simulink model "moban1"  (R2022b)
settings: Solver=VariableStepAuto  StartTime=0.0  StopTime=4  RelTol=1e-3
InitFcn:
  | clear all;
  | 
  | Step_time=2;  %并网转离网的切换时间
  | Tf=0.0159*0.25 %直流侧电流滤波常数
  | 
  | Vdc_H2=720;   %直流母线电压最大值
  | Vdc_H1=710;   %
  | Udc=700;   %直流母线电压最大值
  | Vdc_L1=690;
  | Vdc_L2=680;   %直流母线电压最小值
  | 
  | %% 并网变流器部分 %%
  | P_grid=100e3;  %变流器额定功率
  | Cg=3227e-6;   %直流母线电容
  | P_grid=100e3;  %变流器额定功率
  | Idc_max=145;   %直流侧最大输出电流
  | %Rg=(720-700)/Idc_max;   %下垂系数
  | Rg=40*(Udc-40)/P_grid;   %下垂系数
  | Igrid_max=72;   %并网逆变器最大充放电电流（交流侧）
  | 
  | %% 蓄电池部分 %%
  | P_ba=50e3;  %变流器额定功率
  | R_ba=40*(Udc-40)/P_ba;
  | %Idc_max_ba=147;   %直流侧最大输出电流
  | %R_ba=(Vdc_L1-Vdc_L2)/P_ba;   %下垂系数
  | Iba_max=50;   %蓄电池恒流充放电电流
  | 
  | %% 光伏部分 %%
  | P_PV=150e3;  %变流器额定功率
  | R_PV=40*(Udc-40)/P_PV;   %下垂系数
  | Idc_max_PV=147;   %直流侧最大输出电流
model workspace (MAT data in the model file):
  C = 0.002
  GP = 1
  GQ = 0.01
  J = 5
  KQ = 0.06
  Kf = 800
  Kv = 577
  L = 0.002
  Ts = 5e-05
  Vdc = 400
  fsw = 20000
  wn = 314.159265359
undefined symbols (not defined in the file): DiscIntNeverNeededParam, Ion, Lithium, sigbuilder_block
libraries: spsCurrentMeasurementLib x8, spsSeriesRLCBranchLib x6, slpidlib x6, spsDiodeLib x4, spsVoltageMeasurementLib x3, spsFirstOrderFilterLib x3, spsabctodq0Lib x3, spsIGBTLib x3, spsThreePhaseSeriesRLCBranchLib x2, spsThreePhaseVIMeasurementLib x2, simulink x2, spsPower3phInstantaneousLib x1
(part 1 of 2)
settings Model: Creator=匡磊  LastModifiedBy=刘明炜
settings DataIOCC: ReturnWorkspaceOutputs=off

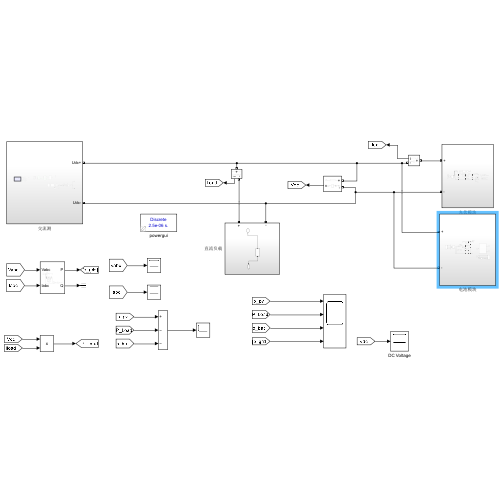
[thumbnail: Simulink's stored preview of the top-level diagram]
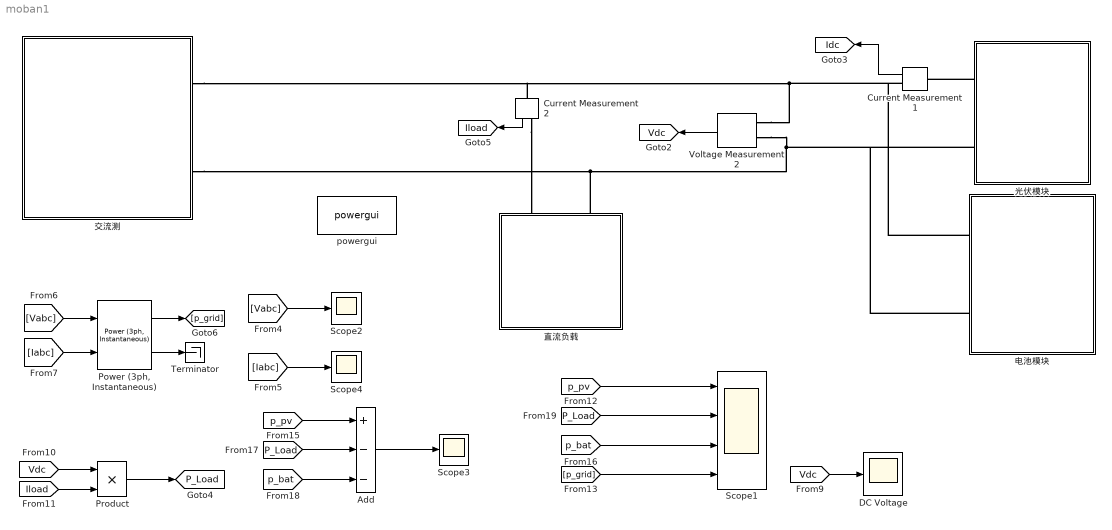
== system moban1 ==
  Add : Sum  Inputs=+--
  Current Measurement1 : spsCurrentMeasurementLib/Current Measurement  PhasorSimulation=off  OutputType=Complex  PSBequivalent=0
  Current Measurement2 : spsCurrentMeasurementLib/Current Measurement  PhasorSimulation=off  OutputType=Complex  PSBequivalent=0
  DC Voltage : Scope
  "Power (3ph, Instantaneous)" : spsPower3phInstantaneousLib/Power (3ph, Instantaneous)
  Product : Product
  Scope1 : Scope  NumInputPorts=4
  Scope2 : Scope
  Scope3 : Scope
  Scope4 : Scope
  Terminator : Terminator
  Voltage Measurement2 : spsVoltageMeasurementLib/Voltage Measurement  PhasorSimulation=off  OutputType=Complex  PSBequivalent=0
  powergui : spspowerguiLib/powergui  Priority=1  SimulationMode=Discrete  SampleTime=2.5e-6  frequency=60  Iterations=50  frequencyindice=0  Pbase=100e6  ErrMax=1e-4  UnitsV=kV  UnitsW=MW  buscounter=0  FunctionMessages=off  echomessages=off  EnableUseOfTLC=off  CurrentSourceSwitches=off  DisableSnubberDevices=off  DisableRonSwitches=off  DisableVfSwitches=off  DisplayEquations=off  AutomaticDiscreteSolvers=off  SolverType=Tustin/Backward Euler (TBE)  Interpol=off  ExternalGateDelay=off  methode=off  Ts=100  x0status=blocks  SPID=on  SwTol=0  HookPort=off  NonlinearTolerance=1e-4  nMaxIteration=100  ContinueOnMaxIteration=off  RestoreLinks=warning  ResistiveCurrentMeasurement=off  Frange=[0:2:500]  Ylog=off  Xlog=on  ShowGrid=off  save=off  variable=ZData  structure=0  ZoomFFT=off  StartTime=0.0  cycles=1  DisplayStyle=1  fundamental=60  FreqAxis=off  MaxFrequency=1000  frequencyindicesteady=1  RmsSteady=1  display=off
  交流测 : Subsystem
  光伏模块 : Subsystem
  电池模块 : Subsystem
  直流负载 : Subsystem
  tag scope: Idc=global, Iload=global, P_Load=global, Vdc=global
  wires:
  [p_pv] -> Scope1/1
  "Power (3ph, Instantaneous)"/1 -> [p_grid]
  [P_Load] -> Scope1/2
  [p_grid] -> Scope1/4
  Add/1 -> Scope3/1
  Current Measurement1/1 -> [Idc]
  [P_Load] -> Add/2
  [p_bat] -> Add/3
  [Vdc] -> DC Voltage/1
  Voltage Measurement2/1 -> [Vdc]
  [Vabc] -> "Power (3ph, Instantaneous)"/1
  [Vdc] -> Product/1
  [Iload] -> Product/2
  [p_pv] -> Add/1
  Product/1 -> [P_Load]
  Current Measurement2/1 -> [Iload]
  [p_bat] -> Scope1/3
  "Power (3ph, Instantaneous)"/2 -> Terminator/1
  [Iabc] -> "Power (3ph, Instantaneous)"/2
  [Vabc] -> Scope2/1
  [Iabc] -> Scope4/1
  connections:
  Voltage Measurement2/LConn1 -- Current Measurement2/LConn1 -- 交流测/LConn1 -- 电池模块/LConn1 -- Current Measurement1/RConn1
  交流测/LConn2 -- 直流负载/LConn2 -- 电池模块/LConn2 -- 光伏模块/LConn2 -- Voltage Measurement2/LConn2
  光伏模块/LConn1 -- Current Measurement1/LConn1
  Current Measurement2/RConn1 -- 直流负载/LConn1

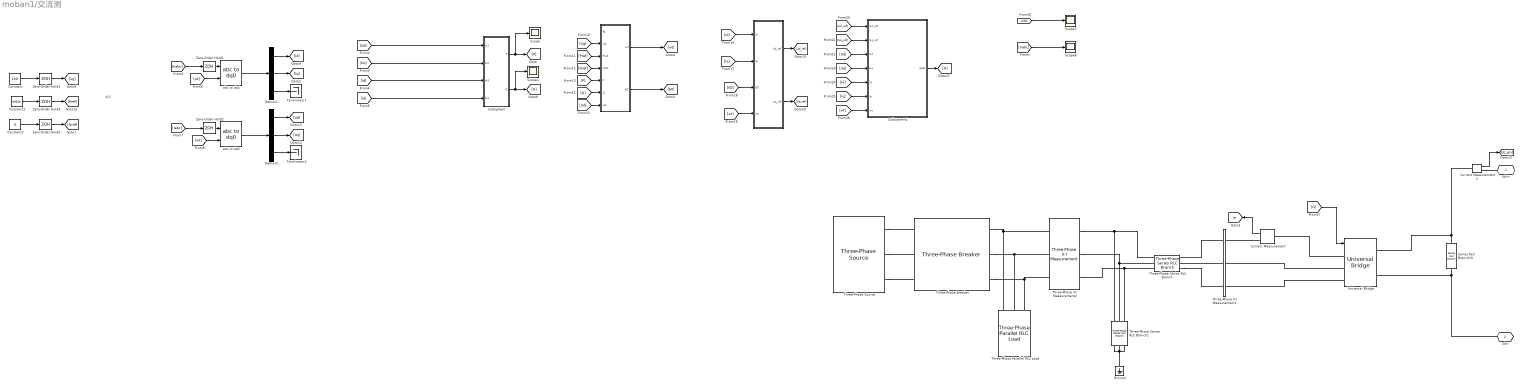
== system moban1/交流测 ==
  note: 给定
  "  " : Subsystem
  "   " : Subsystem
  Constant : Constant  Value=150
  Constant1 : Constant  Value=50000
  Constant2 : Constant  Value=0
  Current Measurement : spsCurrentMeasurementLib/Current Measurement  PhasorSimulation=off  OutputType=Complex  PSBequivalent=0
  Current Measurement1 : spsCurrentMeasurementLib/Current Measurement  PhasorSimulation=off  OutputType=Complex  PSBequivalent=0
  Demux1 : Demux  Outputs=3
  Demux2 : Demux  Outputs=3
  Ground : spsGroundLib/Ground  LConnTagsString=a
  Scope{,1,6..7} (4 alike) : Scope
  Series RLC Branch10 : spsSeriesRLCBranchLib/Series RLC Branch  LConnTagsString=__new0  RConnTagsString=__new0  BranchType=C  Resistance=0.001  Inductance=1e-3  SetiL0=off  InitialCurrent=0  Capacitance=Cg  Setx0=off  InitialVoltage=700  Measurements=None
  Subsystem : Subsystem
  Subsystem1 : Subsystem
  Terminator1 : Terminator
  Terminator2 : Terminator
  Three-Phase Parallel RLC Load : spsThreePhaseParallelRLCLoadLib/Three-Phase Parallel RLC Load  LConnTagsString=A|B|C  RConnTagsString=N  Configuration=Y (neutral)  NominalVoltage=380  Vabc=[1e3 1e3 1e3]  Vabcp=[1e3 1e3 1e3]  NominalFrequency=50  UnbalancedPower=off  ActivePower=50e3  InductivePower=0  CapacitivePower=0  Pabc=[10e3 9e3 11e3]  QLabc=[100 90 110]  QCabc=[100 90 110]  Pabcp=[10e3 9e3 11e3]  QLabcp=[100 90 110]  QCabcp=[100 90 110]  Measurements=None  LoadType=constant Z
  Three-Phase Series RLC Branch : spsThreePhaseSeriesRLCBranchLib/Three-Phase Series RLC Branch  LConnTagsString=A|B|C  RConnTagsString=A|B|C  BranchType=RL  Resistance=0  Inductance=7e-3  Capacitance=1e-6  Measurements=None
  Three-Phase Series RLC Branch1 : spsThreePhaseSeriesRLCBranchLib/Three-Phase Series RLC Branch  LConnTagsString=A|B|C  RConnTagsString=A|B|C  BranchType=RC  Resistance=1  Inductance=7e-3  Capacitance=1500e-6  Measurements=None
  Three-Phase V-I Measurement1 : spsThreePhaseVIMeasurementLib/Three-Phase V-I Measurement  VoltageMeasurement=no  SetLabelV=on  LabelV=Vabc  Vpu=off  VpuLL=off  CurrentMeasurement=yes  SetLabelI=on  LabelI=Iabc  Ipu=off  Pbase=100e6  Vbase=500e3  OutputType=Complex  PhasorSimulation=off  PSBequivalent=0
  Three-Phase V-I Measurement2 : spsThreePhaseVIMeasurementLib/Three-Phase V-I Measurement  VoltageMeasurement=phase-to-ground  SetLabelV=on  LabelV=Vabc  Vpu=off  VpuLL=off  CurrentMeasurement=no  SetLabelI=off  LabelI=Iabc1  Ipu=off  Pbase=100e6  Vbase=500e3  OutputType=Complex  PhasorSimulation=off  PSBequivalent=0
  Three-Phase Breaker : spsThreePhaseBreakerLib/Three-Phase Breaker  InitialState=closed  SwitchA=on  SwitchB=on  SwitchC=on  SwitchTimes=[1 1.5]  External=off  BreakerResistance=0.001  SnubberResistance=10e5  SnubberCapacitance=inf  Measurements=None
  Three-Phase Source : spsThreePhaseSourceLib/Three-Phase Source  InternalConnection=Y  VoltagePhases=off  Voltage=380  PhaseAngle=0  Voltage_phases=[25e3 25e3 25e3]/sqrt(3)  PhaseAngles_phases=[0 -120 +120]  Frequency=50  NonIdealSource=on  SpecifyImpedance=off  Resistance=0.001e-3  Inductance=0.001e-9  ShortCircuitLevel=100e6  BaseVoltage=380  XRratio=7  BusType=swing  Pref=10e3  Qref=0  Prefabc=[10e3, 10e3, 10e3]  Qrefabc=[0, 0, 0]  Qmin=-inf  Qmax=inf
  Universal Bridge : spsUniversalBridgeLib/Universal Bridge  Arms=3  SnubberResistance=1e5  SnubberCapacitance=inf  Device=IGBT / Diodes  Ron=1e-3  Lon=0  ForwardVoltages="[  0  0  ]"  ForwardVoltage=0  GTOparameters=[ 10e-6 , 20e-6 ]  IGBTparameters=[ 1e-6 , 2e-6 ]  Measurements=None  Measurements_2=None  converterType=Rectifier
  Zero-Order Hold{1..5} (5 alike) : ZeroOrderHold  SampleTime=1/fsw
  abc to dq1 : spsabctodq0Lib/abc to dq0  Alignment=90 degrees behind phase A axis
  abc to dq2 : spsabctodq0Lib/abc to dq0  Alignment=90 degrees behind phase A axis
  Udc+ : PMIOPort  Side=Left
  Udc- : PMIOPort  Port=2  Side=Left
  tag scope: Ia=global, Idc_grid=global
  wires:
  Current Measurement1/1 -> [Idc_grid]
  Current Measurement/1 -> [Ia]
  Demux1/3 -> Terminator1/1
  Zero-Order Hold1/1 -> abc to dq1/1
  Demux2/3 -> Terminator2/1
  abc to dq1/1 -> Demux1/1
  Zero-Order Hold2/1 -> abc to dq2/1
  Demux1/2 -> [Iq]
  abc to dq2/1 -> Demux2/1
  Demux2/1 -> [Ud]
  Demux1/1 -> [Id]
  Demux2/2 -> [Uq]
  [Ud] -> Subsystem/1(In1)
  [Uq] -> Subsystem/2(In2)
  [Id] -> Subsystem/3(In3)
  [Iq] -> Subsystem/4(In4)
  [Vabc] -> Zero-Order Hold1/1
  [Iabc] -> Zero-Order Hold2/1
  "  "/2(E0) -> [E0]
  "  "/1(wt) -> [wt]
  [wt] -> abc to dq2/2
  [wt] -> abc to dq1/2
  Zero-Order Hold3/1 -> [Ug]
  Zero-Order Hold5/1 -> [Qref]
  Zero-Order Hold4/1 -> [Pref]
  Constant/1 -> Zero-Order Hold3/1
  Constant1/1 -> Zero-Order Hold4/1
  Constant2/1 -> Zero-Order Hold5/1
  [Ug] -> "  "/2(Ug)
  [Pref] -> "  "/3(Pref)
  [Qref] -> "  "/4(Qref)
  Subsystem/1(P) -> Scope/1, [P]
  [P] -> "  "/5(P)
  [Q] -> "  "/6(Q)
  [Ud] -> "  "/7(Ud)
  "   "/1(Ud_ref) -> [Ud_ref]
  "   "/2(Uq_ref) -> [Uq_ref]
  [Id] -> "   "/1(Id)
  [Iq] -> "   "/2(Iq)
  [E0] -> "   "/3(E0)
  [wt] -> "   "/4(wt)
  Subsystem1/1(gate) -> [G]
  [Ud_ref] -> Subsystem1/1(Ud_ref)
  [Uq_ref] -> Subsystem1/2(Uq_ref)
  [Ud] -> Subsystem1/3(Ud)
  [Uq] -> Subsystem1/4(Uq)
  [Id] -> Subsystem1/5(Id)
  [Iq] -> Subsystem1/6(Iq)
  [wt] -> Subsystem1/7(wt)
  [G] -> Universal Bridge/1
  [Vabc] -> Scope6/1
  [Vdc] -> Scope7/1
  Subsystem/2(Q) -> Scope1/1, [Q]
  connections:
  Udc-/RConn1 -- Universal Bridge/RConn2 -- Series RLC Branch10/RConn1
  Series RLC Branch10/LConn1 -- Current Measurement1/LConn1 -- Universal Bridge/RConn1
  Ground/LConn1 -- Three-Phase Series RLC Branch1/RConn1 -- Three-Phase Series RLC Branch1/RConn3 -- Three-Phase Series RLC Branch1/RConn2
  Three-Phase Breaker/RConn2 -- Three-Phase Parallel RLC Load/LConn2 -- Three-Phase V-I Measurement2/LConn2
  Three-Phase V-I Measurement2/RConn1 -- Three-Phase Series RLC Branch1/LConn1 -- Three-Phase Series RLC Branch/LConn1
  Three-Phase Breaker/RConn1 -- Three-Phase Parallel RLC Load/LConn1 -- Three-Phase V-I Measurement2/LConn1
  Three-Phase V-I Measurement2/RConn3 -- Three-Phase Series RLC Branch1/LConn3 -- Three-Phase Series RLC Branch/LConn3
  Three-Phase V-I Measurement2/RConn2 -- Three-Phase Series RLC Branch1/LConn2 -- Three-Phase Series RLC Branch/LConn2
  Three-Phase Breaker/RConn3 -- Three-Phase V-I Measurement2/LConn3 -- Three-Phase Parallel RLC Load/LConn3
  Three-Phase Series RLC Branch/RConn3 -- Three-Phase V-I Measurement1/RConn3
  Three-Phase Source/RConn1 -- Three-Phase Breaker/LConn1
  Three-Phase V-I Measurement1/LConn1 -- Current Measurement/RConn1
  Current Measurement1/RConn1 -- Udc+/RConn1
  Three-Phase V-I Measurement1/RConn2 -- Three-Phase Series RLC Branch/RConn2
  Three-Phase Source/RConn3 -- Three-Phase Breaker/LConn3
  Three-Phase Source/RConn2 -- Three-Phase Breaker/LConn2
  Three-Phase V-I Measurement1/RConn1 -- Three-Phase Series RLC Branch/RConn1
  Universal Bridge/LConn1 -- Current Measurement/LConn1
  Universal Bridge/LConn2 -- Three-Phase V-I Measurement1/LConn2
  Universal Bridge/LConn3 -- Three-Phase V-I Measurement1/LConn3

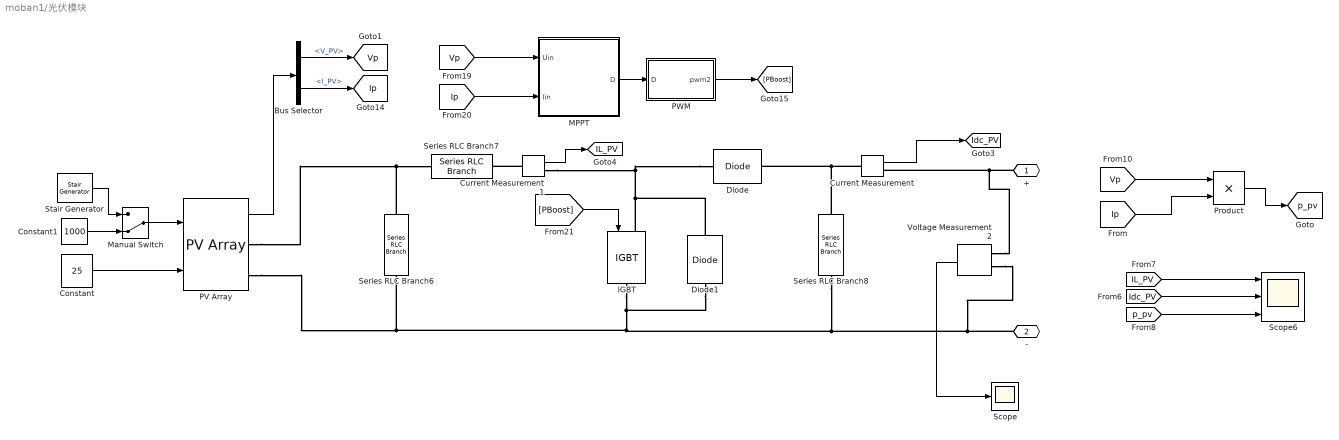
== system moban1/光伏模块 ==
  Bus Selector : BusSelector  OutputSignals=V_PV,I_PV
  Constant : Constant  Value=25
  Constant1 : Constant  Value=1000
  Current Measurement : spsCurrentMeasurementLib/Current Measurement  PhasorSimulation=off  OutputType=Complex  PSBequivalent=0
  Current Measurement1 : spsCurrentMeasurementLib/Current Measurement  PhasorSimulation=off  OutputType=Complex  PSBequivalent=0
  Diode : spsDiodeLib/Diode  Ron=0.001  Lon=0  Vf=0.8  IC=0  UseSnubber=off  Rs=500  Cs=250e-9  Measurements=off
  Diode1 : spsDiodeLib/Diode  Ron=0.001  Lon=0  Vf=0.8  IC=0  UseSnubber=off  Rs=500  Cs=250e-9  Measurements=off
  IGBT : spsIGBTLib/IGBT  Ron=0.001  Lon=0  Vf=1  Tf=1e-6  Tt=2e-6  IC=0  Rs=1e5  Cs=inf  Measurements=off
  MPPT : Subsystem
  Manual Switch : ManualSwitch  CurrentSetting=0
  PV Array : spsPVArrayLib/PV Array  Npar=50  Nser=15  PlotType=array @ 1000 W/m2 & specified temperatures  S_vec="[ 1000  500  100 ]"  Temp_C_vec="[ 45 25  ]"  ModuleName=User-defined  PlotWhenSelected=off  Pm=200  Ncell=60  Voc=36.3  Isc=6.81  Vm=32  Im=6.25  beta_Voc_pc=-0.36099  alpha_Isc_pc=0.102  beta_Voc=-0.13104  alpha_Isc=0.0069462  IL=6.81  I0=1.035e-10  nI=1.0006  Rsh=114.2861  Rs=0.26023  RobustModel=off  RobustCellTemperature=313.3991  BAL=off  Tc=1e-6  Tfilter=5e-5
  PWM : Subsystem
  Product : Product
  Scope : Scope
  Scope6 : Scope  NumInputPorts=3
  Series RLC Branch6 : spsSeriesRLCBranchLib/Series RLC Branch  LConnTagsString=__new0  RConnTagsString=__new0  BranchType=RC  Resistance=1e-3  Inductance=1e-3  SetiL0=off  InitialCurrent=0  Capacitance=1e-3  Setx0=off  InitialVoltage=0  Measurements=None
  Series RLC Branch7 : spsSeriesRLCBranchLib/Series RLC Branch  LConnTagsString=__new0  RConnTagsString=__new0  BranchType=L  Resistance=1  Inductance=1.45e-3  SetiL0=off  InitialCurrent=0  Capacitance=1e-3  Setx0=off  InitialVoltage=0  Measurements=None
  Series RLC Branch8 : spsSeriesRLCBranchLib/Series RLC Branch  LConnTagsString=__new0  RConnTagsString=__new0  BranchType=C  Resistance=1  Inductance=1e-3  SetiL0=off  InitialCurrent=0  Capacitance=3227e-6  Setx0=off  InitialVoltage=700  Measurements=None
  Stair Generator : spsStairGeneratorLib/Stair Generator  t=[0, 0.5, 1, 1.5]  e=[1000, 800, 1200, 800]  Ts=0
  Voltage Measurement2 : spsVoltageMeasurementLib/Voltage Measurement  PhasorSimulation=off  OutputType=Complex  PSBequivalent=0
  + : PMIOPort  Side=Left
  - : PMIOPort  Port=2  Side=Left
  tag scope: IL_PV=global, Idc_PV=global, Ip=global, Vp=global, p_pv=global
  wires:
  Stair Generator/1 -> Manual Switch/1
  Manual Switch/1 -> PV Array/1
  [Ip] -> MPPT/2(Iin)
  Bus Selector/1 -> [Vp]  "<V_PV>"
  [Vp] -> Product/1
  [Ip] -> Product/2
  Constant/1 -> PV Array/2
  Current Measurement/1 -> [Idc_PV]
  [PBoost] -> IGBT/1
  PWM/1(pwm2) -> [PBoost]
  Constant1/1 -> Manual Switch/2
  Voltage Measurement2/1 -> Scope/1
  [p_pv] -> Scope6/3
  [Vp] -> MPPT/1(Uin)
  [IL_PV] -> Scope6/1
  PV Array/1 -> Bus Selector/1
  Current Measurement1/1 -> [IL_PV]
  [Idc_PV] -> Scope6/2
  Product/1 -> [p_pv]
  MPPT/1(D) -> PWM/1(D)
  Bus Selector/2 -> [Ip]  "<I_PV>"
  connections:
  Current Measurement/RConn1 -- +/RConn1 -- Voltage Measurement2/LConn1
  PV Array/RConn2 -- Series RLC Branch6/RConn1 -- Diode1/LConn1 -- IGBT/RConn1 -- -/RConn1 -- Voltage Measurement2/LConn2 -- Series RLC Branch8/RConn1
  Diode/LConn1 -- IGBT/LConn1 -- Diode1/RConn1 -- Current Measurement1/RConn1
  PV Array/RConn1 -- Series RLC Branch6/LConn1 -- Series RLC Branch7/LConn1
  Current Measurement/LConn1 -- Series RLC Branch8/LConn1 -- Diode/RConn1
  Current Measurement1/LConn1 -- Series RLC Branch7/RConn1

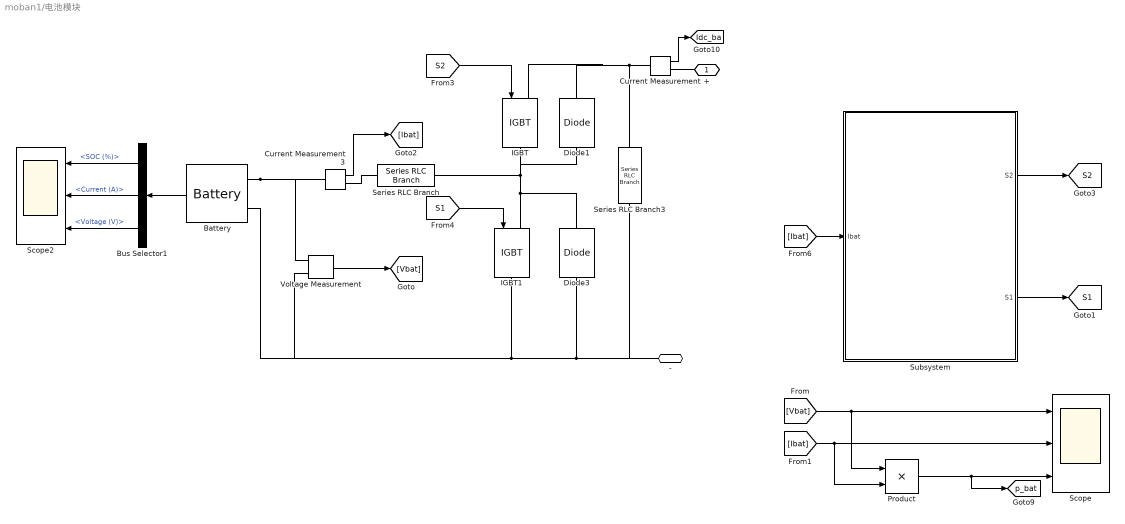
== system moban1/电池模块 ==
  Battery : spsBatteryLib/Battery  BatType=Lithium-Ion  ShowTempParam=off  ThermalPreset=no  ShowAgeParam=off  NomV=300  NomQ=100  SOC=70  Batt_Tr=0.1  PresetModel=on  MaxQ=100  MinV=225  FullV=349.1961  Dis_rate=43.4783  R=0.03  Normal_OP=90.4348  expZone="[324.1158      4.913043]"  current=[6.5 13 32.5]  Units=Time  Tci=20  NomT=20  T2=-30  MaxQ2=4.8  FullV2=7.1  Normal_OP2=5.655  expZone2="[6.58           1]"  Rca=0.6  ti=2000  Dp=0  Neq0=0  Tsim=1e6  Ta1=25  Qeol=5.4*0.9  Reol=0.013333*1.2  Char_age=[2.3478, 3]  Dis_age=[2.3478, 10]  N1=1500  N2=10500  N3=1000  N4=1400  Ta2=45  N5=950
      settings: LibrarySourceBlock=electricdrivelib/Extra Sources/Battery
  Bus Selector1 : BusSelector  OutputSignals=SOC (%),Current (A),Voltage (V)
  Current Measurement : spsCurrentMeasurementLib/Current Measurement  PhasorSimulation=off  OutputType=Complex  PSBequivalent=0
  Current Measurement3 : spsCurrentMeasurementLib/Current Measurement  PhasorSimulation=off  OutputType=Complex  PSBequivalent=0
  Diode1 : spsDiodeLib/Diode  Ron=0.001  Lon=0  Vf=0.8  IC=0  UseSnubber=off  Rs=500  Cs=250e-9  Measurements=off
  Diode3 : spsDiodeLib/Diode  Ron=0.001  Lon=0  Vf=0.8  IC=0  UseSnubber=off  Rs=500  Cs=250e-9  Measurements=off
  IGBT : spsIGBTLib/IGBT  Ron=0.001  Lon=0  Vf=1  Tf=1e-6  Tt=2e-6  IC=0  Rs=1e5  Cs=inf  Measurements=off
  IGBT1 : spsIGBTLib/IGBT  Ron=0.001  Lon=0  Vf=1  Tf=1e-6  Tt=2e-6  IC=0  Rs=1e5  Cs=inf  Measurements=off
  Product : Product
  Scope : Scope  NumInputPorts=3
  Scope2 : Scope  NumInputPorts=3
  Series RLC Branch : spsSeriesRLCBranchLib/Series RLC Branch  LConnTagsString=__new0  RConnTagsString=__new0  BranchType=L  Resistance=1  Inductance=0.002  SetiL0=off  InitialCurrent=0  Capacitance=1e-6  Setx0=off  InitialVoltage=0  Measurements=None
  Series RLC Branch3 : spsSeriesRLCBranchLib/Series RLC Branch  LConnTagsString=__new0  RConnTagsString=__new0  BranchType=C  Resistance=1  Inductance=1e-3  SetiL0=off  InitialCurrent=0  Capacitance=220e-6  Setx0=off  InitialVoltage=0  Measurements=None
  Subsystem : Subsystem
  Voltage Measurement : spsVoltageMeasurementLib/Voltage Measurement  PhasorSimulation=off  OutputType=Complex  PSBequivalent=0
  + : PMIOPort  Side=Left
  - : PMIOPort  Port=2  Side=Left
  tag scope: Idc_ba=global, S1=global, S2=global, p_bat=global
  wires:
  Current Measurement/1 -> [Idc_ba]
  Bus Selector1/1 -> Scope2/1  "<SOC (%)>"
  Current Measurement3/1 -> [Ibat]
  Subsystem/1(S2) -> [S2]
  [Ibat] -> Subsystem/1(Ibat)
  Subsystem/2(S1) -> [S1]
  [Vbat] -> Scope/1, Product/1
  Voltage Measurement/1 -> [Vbat]
  Bus Selector1/2 -> Scope2/2  "<Current (A)>"
  [S2] -> IGBT/1
  Battery/1 -> Bus Selector1/1
  [Ibat] -> Scope/2, Product/2
  Bus Selector1/3 -> Scope2/3  "<Voltage (V)>"
  [S1] -> IGBT1/1
  Product/1 -> [p_bat], Scope/3
  connections:
  Diode3/RConn1 -- IGBT1/LConn1 -- Series RLC Branch/RConn1 -- Diode1/LConn1 -- IGBT/RConn1
  Battery/LConn1 -- Voltage Measurement/LConn1 -- Current Measurement3/LConn1
  Current Measurement/LConn1 -- Series RLC Branch3/LConn1 -- Diode1/RConn1 -- IGBT/LConn1
  IGBT1/RConn1 -- Voltage Measurement/LConn2 -- Battery/LConn2 -- Series RLC Branch3/RConn1 -- -/RConn1 -- Diode3/LConn1
  +/RConn1 -- Current Measurement/RConn1
  Current Measurement3/RConn1 -- Series RLC Branch/LConn1

== system moban1/直流负载 ==
  Series RLC Load1 : spsSeriesRLCLoadLib/Series RLC Load  LConnTagsString=a  RConnTagsString=__new0  NominalVoltage=700  NominalFrequency=50  ActivePower=110e3  InductivePower=0  CapacitivePower=0  Setx0=off  InitialVoltage=0  SetiL0=off  InitialCurrent=0  Measurements=None  LoadType=constant Z
  + : PMIOPort  Side=Left
  - : PMIOPort  Port=2  Side=Left
  connections:
  Series RLC Load1/RConn1 -- -/RConn1
  +/RConn1 -- Series RLC Load1/LConn1

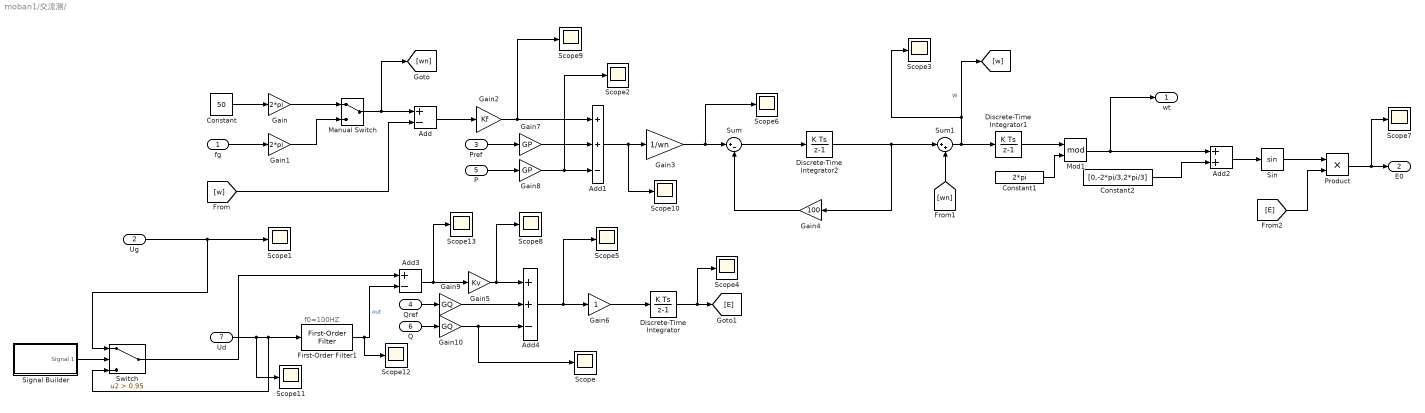
== system moban1/交流测/   ==
  note: f0=100HZ
  note: w
  fg : Inport
  Ug : Inport  Port=2
  Pref : Inport  Port=3
  Qref : Inport  Port=4
  P : Inport  Port=5
  Q : Inport  Port=6
  Ud : Inport  Port=7
  Add : Sum  Inputs=+-
  Add1 : Sum  Inputs=++-
  Add2 : Sum
  Add3 : Sum  Inputs=+-
  Add4 : Sum  Inputs=++-
  Constant : Constant  Value=50
  Constant1 : Constant  Value=2*pi
  Constant2 : Constant  Value=[0,-2*pi/3,2*pi/3]
  Discrete-Time Integrator : DiscreteIntegrator  gainval=KQ  SampleTime=1/fsw  ICPrevOutput=DiscIntNeverNeededParam  ICPrevScaledInput=DiscIntNeverNeededParam
  Discrete-Time Integrator1 : DiscreteIntegrator  SampleTime=1/fsw  ICPrevOutput=DiscIntNeverNeededParam  ICPrevScaledInput=DiscIntNeverNeededParam
  Discrete-Time Integrator2 : DiscreteIntegrator  gainval=1/J  SampleTime=1/fsw  ICPrevOutput=DiscIntNeverNeededParam  ICPrevScaledInput=DiscIntNeverNeededParam
  First-Order Filter1 : spsFirstOrderFilterLib/First-Order Filter  FilterType=Lowpass  Tc=10e-3  Ts=1/fsw  Initialize=on  Vac_Init=[0, 0, 10]  Vdc_Init=0  PlotResponse=off  FreqRange="[0,  200,  1]"
  Gain : Gain  Gain=2*pi
  Gain1 : Gain  Gain=2*pi
  Gain10 : Gain  Gain=GQ
  Gain2 : Gain  Gain=Kf
  Gain3 : Gain  Gain=1/wn
  Gain4 : Gain  Gain=100
  Gain5 : Gain  Gain=Kv
  Gain6 : Gain
  Gain7 : Gain  Gain=GP
  Gain8 : Gain  Gain=GP
  Gain9 : Gain  Gain=GQ
  Manual Switch : ManualSwitch
  Mod1 : Math  Operator=mod
  Product : Product
  Scope{,1..13} (14 alike) : Scope
  Signal Builder : Subsystem  Tag=STV Subsys  LoadFcn=sigbuilder_block('load');  StartFcn=sigbuilder_block('start');  StopFcn=sigbuilder_block('stop');  ClipboardFcn=sigbuilder_block('clipboard');  mask(Sigbuilder block){tuvar=[0:10]}
      mask help: Simulink:masks:SigbuilderBlock_MD
      mask init:
      | if ~strcmp(get_param(bdroot(gcbh),'SimulationStatus'),'stopped') tuvar = sigbuilder_block('maskInit'); end
      settings: CopyFcn=sigbuilder_block('copy');  DeleteFcn=sigbuilder_block('delete');  ModelCloseFcn=sigbuilder_block('modelClose');  PreSaveFcn=sigbuilder_block('preSave');  PauseFcn=sigbuilder_block('pause');  ContinueFcn=sigbuilder_block('continue');  NameChangeFcn=sigbuilder_block('namechange');  OpenFcn=sigbuilder_block('open',[437.6 199.2 550.4 400 ]);  CloseFcn=sigbuilder_block('close');
      mask Display: plot(0, 0, 100, 100,[2, 2, 32, 32, 2], [68, 8, 8, 68, 68],[32, 2], [38, 38], [32, 19, 2],[53, 60, 44], [32, 17, 17, 2],[16, 16, 31, 31]);txt = getActiveGroup(gcbh);text(2, 100, txt,'verticalAlignment', 'top');
  Sin : Trigonometry
  Sum : Sum  Inputs=|+-
  Sum1 : Sum  Inputs=|++
  Switch : Switch  Criteria=u2 > Threshold  Threshold=0.95  SaturateOnIntegerOverflow=off  InputSameDT=off
  wt : Outport
  E0 : Outport  Port=2
  wires:
  Ug/1 -> Switch/1, Scope1/1
  Gain3/1 -> Scope6/1, Sum/1
  Gain2/1 -> Scope9/1, Add1/1
  Product/1 -> Scope7/1, E0/1
  Add/1 -> Gain2/1
  [E] -> Product/2
  Add4/1 -> Scope5/1, Gain6/1
  Mod1/1 -> wt/1, Add2/1
  Sum1/1 -> Discrete-Time Integrator1/1, Scope3/1, [w]
  fg/1 -> Gain1/1
  Constant2/1 -> Add2/2
  First-Order Filter1/1 -> Scope12/1, Add3/2  "out"
  Constant/1 -> Gain/1
  Sin/1 -> Product/1
  Add2/1 -> Sin/1
  Gain4/1 -> Sum/2
  P/1 -> Gain8/1
  Gain/1 -> Manual Switch/1
  Gain1/1 -> Manual Switch/2
  Discrete-Time Integrator2/1 -> Gain4/1, Sum1/1
  Constant1/1 -> Mod1/2
  Gain5/1 -> Scope8/1, Add4/1
  Q/1 -> Gain10/1
  Manual Switch/1 -> [wn], Add/1
  Pref/1 -> Gain7/1
  Add1/1 -> Scope10/1, Gain3/1
  Add3/1 -> Scope13/1, Gain5/1
  Gain6/1 -> Discrete-Time Integrator/1
  Qref/1 -> Gain9/1
  [wn] -> Sum1/2
  Sum/1 -> Discrete-Time Integrator2/1
  Discrete-Time Integrator/1 -> Scope4/1, [E]
  Discrete-Time Integrator1/1 -> Mod1/1
  [w] -> Add/2
  Gain7/1 -> Add1/2
  Gain8/1 -> Scope2/1, Add1/3
  Gain9/1 -> Add4/2
  Gain10/1 -> Scope/1, Add4/3
  Ud/1 -> Scope11/1, Switch/3, First-Order Filter1/1
  Signal Builder/1(Signal 1) -> Switch/2
  Switch/1 -> Add3/1

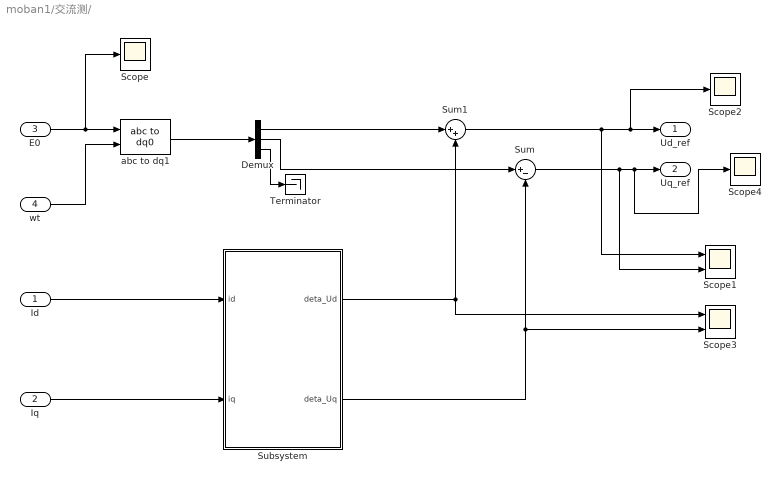
== system moban1/交流测/    ==
  Id : Inport
  Iq : Inport  Port=2
  E0 : Inport  Description=Cont  Port=3
  wt : Inport  Port=4
  Demux : Demux  Outputs=3
  Scope : Scope
  Scope1 : Scope  NumInputPorts=2
  Scope2 : Scope
  Scope3 : Scope  NumInputPorts=2
  Scope4 : Scope
  Subsystem : Subsystem
  Sum : Sum  Inputs=|+-
  Sum1 : Sum  Inputs=|++
  Terminator : Terminator
  abc to dq1 : spsabctodq0Lib/abc to dq0  Alignment=90 degrees behind phase A axis
  Ud_ref : Outport
  Uq_ref : Outport  Port=2
  wires:
  Demux/1 -> Sum1/1
  E0/1 -> Scope/1, abc to dq1/1
  Id/1 -> Subsystem/1(id)
  abc to dq1/1 -> Demux/1
  Subsystem/2(deta_Uq) -> Scope3/2, Sum/2
  Sum1/1 -> Scope2/1, Ud_ref/1, Scope1/1
  wt/1 -> abc to dq1/2
  Demux/2 -> Sum/1
  Subsystem/1(deta_Ud) -> Scope3/1, Sum1/2
  Iq/1 -> Subsystem/2(iq)
  Sum/1 -> Scope4/1, Uq_ref/1, Scope1/2
  Demux/3 -> Terminator/1

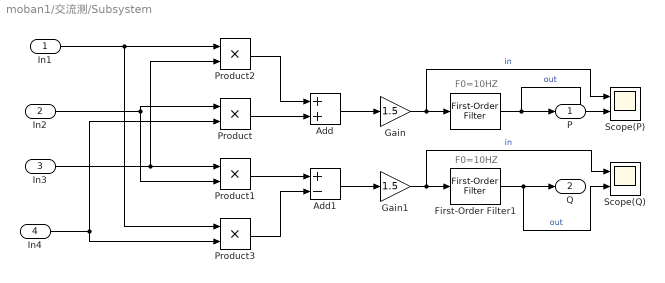
== system moban1/交流测/Subsystem ==
  note: F0=10HZ
  note: F0=10HZ
  In1 : Inport
  In2 : Inport  Port=2
  In3 : Inport  Port=3
  In4 : Inport  Port=4
  " " : spsFirstOrderFilterLib/First-Order Filter  FilterType=Lowpass  Tc=10e-3  Ts=1/fsw  Initialize=on  Vac_Init=[0, 0, 10]  Vdc_Init=0  PlotResponse=off  FreqRange="[0,  200,  1]"
  Add : Sum
  Add1 : Sum  Inputs=+-
  First-Order Filter1 : spsFirstOrderFilterLib/First-Order Filter  FilterType=Lowpass  Tc=10e-3  Ts=1/fsw  Initialize=on  Vac_Init=[0, 0, 10]  Vdc_Init=0  PlotResponse=off  FreqRange="[0,  200,  1]"
  Gain : Gain  Gain=1.5
  Gain1 : Gain  Gain=1.5
  Product{,1..3} (4 alike) : Product
  Scope(P) : Scope  NumInputPorts=2
  Scope(Q) : Scope  NumInputPorts=2
  P : Outport
  Q : Outport  Port=2
  wires:
  First-Order Filter1/1 -> Q/1, Scope(Q)/2  "out"
  Product2/1 -> Add/1
  In1/1 -> Product3/1, Product2/1
  Product3/1 -> Add1/2
  " "/1 -> P/1, Scope(P)/2  "out"
  In4/1 -> Product3/2, Product/2
  Product/1 -> Add/2
  Add1/1 -> Gain1/1
  Product1/1 -> Add1/1
  Add/1 -> Gain/1
  Gain/1 -> " "/1, Scope(P)/1  "in"
  In3/1 -> Product2/2, Product1/1
  Gain1/1 -> First-Order Filter1/1, Scope(Q)/1  "in"
  In2/1 -> Product/1, Product1/2

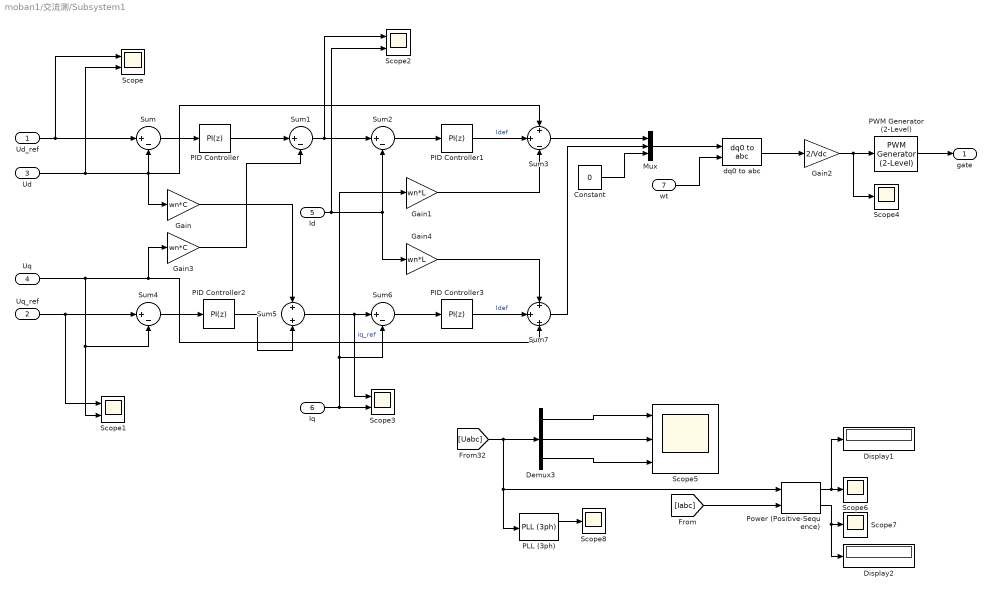
== system moban1/交流测/Subsystem1 ==
  Ud_ref : Inport
  Uq_ref : Inport  Port=2
  Ud : Inport  Port=3
  Uq : Inport  Port=4
  Id : Inport  Port=5
  Iq : Inport  Port=6
  wt : Inport  Port=7
  Constant : Constant  Value=0
  Demux3 : Demux  Outputs=3
  Display1 : Display
  Display2 : Display
  Gain : Gain  Gain=wn*C
  Gain1 : Gain  Gain=wn*L
  Gain2 : Gain  Gain=2/Vdc
  Gain3 : Gain  Gain=wn*C
  Gain4 : Gain  Gain=wn*L
  Mux : Mux  Inputs=3
  PID Controller : slpidlib/PID Controller  Controller=PI  Form=Parallel  TimeDomain=Discrete-time  UseExternalTs=off  SampleTime=-1  IntegratorMethod=Forward Euler  FilterMethod=Forward Euler  ControllerParametersSource=internal  P=20  I=100  UseKiTs=off  D=0  N=100  UseFilter=on  TunerSelectOption=Transfer Function Based (PID Tuner App)  InitialConditionSource=internal  InitialConditionForIntegrator=0  InitialConditionForFilter=0  DifferentiatorICPrevScaledInput=0  ExternalReset=none  TrackingMode=off  Kt=1  LimitOutput=off  SatLimitsSource=internal  UpperSaturationLimit=inf  LowerSaturationLimit=-inf  LinearizeAsGain=on  AntiWindupMode=none  Kb=1  LimitIntegrator=off  UpperIntegratorSaturationLimit=inf  LowerIntegratorSaturationLimit=-inf  POutMin=[]  POutMax=[]  IOutMin=[]  IOutMax=[]  DOutMin=[]  DOutMax=[]  NOutMin=[]  NOutMax=[]  SumOutMin=[]  SumOutMax=[]  SaturationOutMin=[]  SaturationOutMax=[]  PParamMin=[]  PParamMax=[]  IParamMin=[]  IParamMax=[]  DParamMin=[]  DParamMax=[]  NParamMin=[]  NParamMax=[]  KbParamMin=[]  KbParamMax=[]  KtParamMin=[]  KtParamMax=[]  KbOutMin=[]  KbOutMax=[]  KtOutMin=[]  KtOutMax=[]  IntegratorOutMin=[]  IntegratorOutMax=[]  FilterOutMin=[]  FilterOutMax=[]  SumI1OutMin=[]  SumI1OutMax=[]  SumI2OutMin=[]  SumI2OutMax=[]  SumI3OutMin=[]  SumI3OutMax=[]  SumI4OutMin=[]  SumI4OutMax=[]  SumDOutMin=[]  SumDOutMax=[]  DifferentiatorOutMin=[]  DifferentiatorOutMax=[]  FilterDiffOutCoefMin=[]  FilterDiffOutCoefMax=[]  ReciprocalOutMin=[]  ReciprocalOutMax=[]  SumDenOutMin=[]  SumDenOutMax=[]  SumNumOutMin=[]  SumNumOutMax=[]  DivideOutMin=[]  DivideOutMax=[]  UdiffTsProdOutMin=[]  UdiffTsProdOutMax=[]  NTsProdOutMin=[]  NTsProdOutMax=[]  UintegralTsProdOutMin=[]  UintegralTsProdOutMax=[]  UngainTsProdOutMin=[]  UngainTsProdOutMax=[]  ClampingZeroOutDataTypeStr=Inherit: Inherit via back propagation  ClampingZeroOutMin=[]  ClampingZeroOutMax=[]  FilterDenConstantOutDataTypeStr=Inherit: Inherit via back propagation  FilterDenConstantOutMin=[]  FilterDenConstantOutMax=[]  PCopyOutDataTypeStr=Inherit: Inherit via back propagation  PCopyOutMin=[]  PCopyOutMax=[]  NCopyOutDataTypeStr=Inherit: Inherit via back propagation  NCopyOutMin=[]  NCopyOutMax=[]  IntegratorContinuousStateAttributes=''  IntegratorStateMustResolveToSignalObject=off  IntegratorRTWStateStorageClass=Auto  FilterContinuousStateAttributes=''  FilterStateMustResolveToSignalObject=off  FilterRTWStateStorageClass=Auto  ParallelPVariant=InternalParameters  IdealPVariant=Disabled  IVariant=InternalParameters  DVariant=Disabled  IntegratorVariant=Discrete  SatVariant=Disabled  AWVariant=Passthrough  PCopyVariant=Disabled  TRVariant=Disabled  FdbkBlocksVariant=Forward  IdealPFdbkVariant=Disabled  SatFdbkVariant=Disabled  DerivativeFilterVariant=Disabled  NVariant=Disabled  NCopyVariant=Disabled_SignalSpec  FilterICVariant=Disabled  IntegratorICVariant=InternalICs  ExternalResetVariant=Disabled  TRSumVariant=Passthrough  SumFdbkVariant=Disabled  SumVariant=Sum_PI  TsampFilterVariant=InternalTs  TsampNgainVariant=Passthrough  TsampIntegralVariant=Passthrough  ExternalSaturationOutDataTypeStr=Inherit: Same as second input
  PID Controller1 : slpidlib/PID Controller  Controller=PI  Form=Parallel  TimeDomain=Discrete-time  UseExternalTs=off  SampleTime=-1  IntegratorMethod=Forward Euler  FilterMethod=Forward Euler  ControllerParametersSource=internal  P=20  I=50  UseKiTs=off  D=0  N=100  UseFilter=on  TunerSelectOption=Transfer Function Based (PID Tuner App)  InitialConditionSource=internal  InitialConditionForIntegrator=0  InitialConditionForFilter=0  DifferentiatorICPrevScaledInput=0  ExternalReset=none  TrackingMode=off  Kt=1  LimitOutput=off  SatLimitsSource=internal  UpperSaturationLimit=inf  LowerSaturationLimit=-inf  LinearizeAsGain=on  AntiWindupMode=none  Kb=1  LimitIntegrator=off  UpperIntegratorSaturationLimit=inf  LowerIntegratorSaturationLimit=-inf  POutMin=[]  POutMax=[]  IOutMin=[]  IOutMax=[]  DOutMin=[]  DOutMax=[]  NOutMin=[]  NOutMax=[]  SumOutMin=[]  SumOutMax=[]  SaturationOutMin=[]  SaturationOutMax=[]  PParamMin=[]  PParamMax=[]  IParamMin=[]  IParamMax=[]  DParamMin=[]  DParamMax=[]  NParamMin=[]  NParamMax=[]  KbParamMin=[]  KbParamMax=[]  KtParamMin=[]  KtParamMax=[]  KbOutMin=[]  KbOutMax=[]  KtOutMin=[]  KtOutMax=[]  IntegratorOutMin=[]  IntegratorOutMax=[]  FilterOutMin=[]  FilterOutMax=[]  SumI1OutMin=[]  SumI1OutMax=[]  SumI2OutMin=[]  SumI2OutMax=[]  SumI3OutMin=[]  SumI3OutMax=[]  SumI4OutMin=[]  SumI4OutMax=[]  SumDOutMin=[]  SumDOutMax=[]  DifferentiatorOutMin=[]  DifferentiatorOutMax=[]  FilterDiffOutCoefMin=[]  FilterDiffOutCoefMax=[]  ReciprocalOutMin=[]  ReciprocalOutMax=[]  SumDenOutMin=[]  SumDenOutMax=[]  SumNumOutMin=[]  SumNumOutMax=[]  DivideOutMin=[]  DivideOutMax=[]  UdiffTsProdOutMin=[]  UdiffTsProdOutMax=[]  NTsProdOutMin=[]  NTsProdOutMax=[]  UintegralTsProdOutMin=[]  UintegralTsProdOutMax=[]  UngainTsProdOutMin=[]  UngainTsProdOutMax=[]  ClampingZeroOutDataTypeStr=Inherit: Inherit via back propagation  ClampingZeroOutMin=[]  ClampingZeroOutMax=[]  FilterDenConstantOutDataTypeStr=Inherit: Inherit via back propagation  FilterDenConstantOutMin=[]  FilterDenConstantOutMax=[]  PCopyOutDataTypeStr=Inherit: Inherit via back propagation  PCopyOutMin=[]  PCopyOutMax=[]  NCopyOutDataTypeStr=Inherit: Inherit via back propagation  NCopyOutMin=[]  NCopyOutMax=[]  IntegratorContinuousStateAttributes=''  IntegratorStateMustResolveToSignalObject=off  IntegratorRTWStateStorageClass=Auto  FilterContinuousStateAttributes=''  FilterStateMustResolveToSignalObject=off  FilterRTWStateStorageClass=Auto  ParallelPVariant=InternalParameters  IdealPVariant=Disabled  IVariant=InternalParameters  DVariant=Disabled  IntegratorVariant=Discrete  SatVariant=Disabled  AWVariant=Passthrough  PCopyVariant=Disabled  TRVariant=Disabled  FdbkBlocksVariant=Forward  IdealPFdbkVariant=Disabled  SatFdbkVariant=Disabled  DerivativeFilterVariant=Disabled  NVariant=Disabled  NCopyVariant=Disabled_SignalSpec  FilterICVariant=Disabled  IntegratorICVariant=InternalICs  ExternalResetVariant=Disabled  TRSumVariant=Passthrough  SumFdbkVariant=Disabled  SumVariant=Sum_PI  TsampFilterVariant=InternalTs  TsampNgainVariant=Passthrough  TsampIntegralVariant=Passthrough  ExternalSaturationOutDataTypeStr=Inherit: Same as second input
  PID Controller2 : slpidlib/PID Controller  Controller=PI  Form=Parallel  TimeDomain=Discrete-time  UseExternalTs=off  SampleTime=-1  IntegratorMethod=Forward Euler  FilterMethod=Forward Euler  ControllerParametersSource=internal  P=20  I=100  UseKiTs=off  D=0  N=100  UseFilter=on  TunerSelectOption=Transfer Function Based (PID Tuner App)  InitialConditionSource=internal  InitialConditionForIntegrator=0  InitialConditionForFilter=0  DifferentiatorICPrevScaledInput=0  ExternalReset=none  TrackingMode=off  Kt=1  LimitOutput=off  SatLimitsSource=internal  UpperSaturationLimit=inf  LowerSaturationLimit=-inf  LinearizeAsGain=on  AntiWindupMode=none  Kb=1  LimitIntegrator=off  UpperIntegratorSaturationLimit=inf  LowerIntegratorSaturationLimit=-inf  POutMin=[]  POutMax=[]  IOutMin=[]  IOutMax=[]  DOutMin=[]  DOutMax=[]  NOutMin=[]  NOutMax=[]  SumOutMin=[]  SumOutMax=[]  SaturationOutMin=[]  SaturationOutMax=[]  PParamMin=[]  PParamMax=[]  IParamMin=[]  IParamMax=[]  DParamMin=[]  DParamMax=[]  NParamMin=[]  NParamMax=[]  KbParamMin=[]  KbParamMax=[]  KtParamMin=[]  KtParamMax=[]  KbOutMin=[]  KbOutMax=[]  KtOutMin=[]  KtOutMax=[]  IntegratorOutMin=[]  IntegratorOutMax=[]  FilterOutMin=[]  FilterOutMax=[]  SumI1OutMin=[]  SumI1OutMax=[]  SumI2OutMin=[]  SumI2OutMax=[]  SumI3OutMin=[]  SumI3OutMax=[]  SumI4OutMin=[]  SumI4OutMax=[]  SumDOutMin=[]  SumDOutMax=[]  DifferentiatorOutMin=[]  DifferentiatorOutMax=[]  FilterDiffOutCoefMin=[]  FilterDiffOutCoefMax=[]  ReciprocalOutMin=[]  ReciprocalOutMax=[]  SumDenOutMin=[]  SumDenOutMax=[]  SumNumOutMin=[]  SumNumOutMax=[]  DivideOutMin=[]  DivideOutMax=[]  UdiffTsProdOutMin=[]  UdiffTsProdOutMax=[]  NTsProdOutMin=[]  NTsProdOutMax=[]  UintegralTsProdOutMin=[]  UintegralTsProdOutMax=[]  UngainTsProdOutMin=[]  UngainTsProdOutMax=[]  ClampingZeroOutDataTypeStr=Inherit: Inherit via back propagation  ClampingZeroOutMin=[]  ClampingZeroOutMax=[]  FilterDenConstantOutDataTypeStr=Inherit: Inherit via back propagation  FilterDenConstantOutMin=[]  FilterDenConstantOutMax=[]  PCopyOutDataTypeStr=Inherit: Inherit via back propagation  PCopyOutMin=[]  PCopyOutMax=[]  NCopyOutDataTypeStr=Inherit: Inherit via back propagation  NCopyOutMin=[]  NCopyOutMax=[]  IntegratorContinuousStateAttributes=''  IntegratorStateMustResolveToSignalObject=off  IntegratorRTWStateStorageClass=Auto  FilterContinuousStateAttributes=''  FilterStateMustResolveToSignalObject=off  FilterRTWStateStorageClass=Auto  ParallelPVariant=InternalParameters  IdealPVariant=Disabled  IVariant=InternalParameters  DVariant=Disabled  IntegratorVariant=Discrete  SatVariant=Disabled  AWVariant=Passthrough  PCopyVariant=Disabled  TRVariant=Disabled  FdbkBlocksVariant=Forward  IdealPFdbkVariant=Disabled  SatFdbkVariant=Disabled  DerivativeFilterVariant=Disabled  NVariant=Disabled  NCopyVariant=Disabled_SignalSpec  FilterICVariant=Disabled  IntegratorICVariant=InternalICs  ExternalResetVariant=Disabled  TRSumVariant=Passthrough  SumFdbkVariant=Disabled  SumVariant=Sum_PI  TsampFilterVariant=InternalTs  TsampNgainVariant=Passthrough  TsampIntegralVariant=Passthrough  ExternalSaturationOutDataTypeStr=Inherit: Same as second input
  PID Controller3 : slpidlib/PID Controller  Controller=PI  Form=Parallel  TimeDomain=Discrete-time  UseExternalTs=off  SampleTime=-1  IntegratorMethod=Forward Euler  FilterMethod=Forward Euler  ControllerParametersSource=internal  P=20  I=50  UseKiTs=off  D=0  N=100  UseFilter=on  TunerSelectOption=Transfer Function Based (PID Tuner App)  InitialConditionSource=internal  InitialConditionForIntegrator=0  InitialConditionForFilter=0  DifferentiatorICPrevScaledInput=0  ExternalReset=none  TrackingMode=off  Kt=1  LimitOutput=off  SatLimitsSource=internal  UpperSaturationLimit=inf  LowerSaturationLimit=-inf  LinearizeAsGain=on  AntiWindupMode=none  Kb=1  LimitIntegrator=off  UpperIntegratorSaturationLimit=inf  LowerIntegratorSaturationLimit=-inf  POutMin=[]  POutMax=[]  IOutMin=[]  IOutMax=[]  DOutMin=[]  DOutMax=[]  NOutMin=[]  NOutMax=[]  SumOutMin=[]  SumOutMax=[]  SaturationOutMin=[]  SaturationOutMax=[]  PParamMin=[]  PParamMax=[]  IParamMin=[]  IParamMax=[]  DParamMin=[]  DParamMax=[]  NParamMin=[]  NParamMax=[]  KbParamMin=[]  KbParamMax=[]  KtParamMin=[]  KtParamMax=[]  KbOutMin=[]  KbOutMax=[]  KtOutMin=[]  KtOutMax=[]  IntegratorOutMin=[]  IntegratorOutMax=[]  FilterOutMin=[]  FilterOutMax=[]  SumI1OutMin=[]  SumI1OutMax=[]  SumI2OutMin=[]  SumI2OutMax=[]  SumI3OutMin=[]  SumI3OutMax=[]  SumI4OutMin=[]  SumI4OutMax=[]  SumDOutMin=[]  SumDOutMax=[]  DifferentiatorOutMin=[]  DifferentiatorOutMax=[]  FilterDiffOutCoefMin=[]  FilterDiffOutCoefMax=[]  ReciprocalOutMin=[]  ReciprocalOutMax=[]  SumDenOutMin=[]  SumDenOutMax=[]  SumNumOutMin=[]  SumNumOutMax=[]  DivideOutMin=[]  DivideOutMax=[]  UdiffTsProdOutMin=[]  UdiffTsProdOutMax=[]  NTsProdOutMin=[]  NTsProdOutMax=[]  UintegralTsProdOutMin=[]  UintegralTsProdOutMax=[]  UngainTsProdOutMin=[]  UngainTsProdOutMax=[]  ClampingZeroOutDataTypeStr=Inherit: Inherit via back propagation  ClampingZeroOutMin=[]  ClampingZeroOutMax=[]  FilterDenConstantOutDataTypeStr=Inherit: Inherit via back propagation  FilterDenConstantOutMin=[]  FilterDenConstantOutMax=[]  PCopyOutDataTypeStr=Inherit: Inherit via back propagation  PCopyOutMin=[]  PCopyOutMax=[]  NCopyOutDataTypeStr=Inherit: Inherit via back propagation  NCopyOutMin=[]  NCopyOutMax=[]  IntegratorContinuousStateAttributes=''  IntegratorStateMustResolveToSignalObject=off  IntegratorRTWStateStorageClass=Auto  FilterContinuousStateAttributes=''  FilterStateMustResolveToSignalObject=off  FilterRTWStateStorageClass=Auto  ParallelPVariant=InternalParameters  IdealPVariant=Disabled  IVariant=InternalParameters  DVariant=Disabled  IntegratorVariant=Discrete  SatVariant=Disabled  AWVariant=Passthrough  PCopyVariant=Disabled  TRVariant=Disabled  FdbkBlocksVariant=Forward  IdealPFdbkVariant=Disabled  SatFdbkVariant=Disabled  DerivativeFilterVariant=Disabled  NVariant=Disabled  NCopyVariant=Disabled_SignalSpec  FilterICVariant=Disabled  IntegratorICVariant=InternalICs  ExternalResetVariant=Disabled  TRSumVariant=Passthrough  SumFdbkVariant=Disabled  SumVariant=Sum_PI  TsampFilterVariant=InternalTs  TsampNgainVariant=Passthrough  TsampIntegralVariant=Passthrough  ExternalSaturationOutDataTypeStr=Inherit: Same as second input
  PLL (3ph) : spsPLL3phLib/PLL (3ph)  Fmin=45  Par_Init=[0, 50]  ParK=[180, 3200, 1]  TcD=1e-4  MaxRateChangeFreq=12  FilterCutOffFreq=25  Ts=1/fsw  AGC=on
  PWM Generator (2-Level) : spsPWMGenerator2LevelLib/PWM Generator (2-Level)  ModulatorType=Three-phase bridge (6 pulses)  ModulatorMode=Unsynchronized  Fc=fsw  Pc=90  nF=27  MinMax="[ -1  1 ]"  SamplingTechnique=Natural  ModulatingSignals=off  m=0.8  Freq=60  Phase=0  Ts=Ts  ShowCarrierOutport=off
  Power (Positive-Sequence) : spsPowerPositiveSequenceLib/Power (Positive-Sequence)  Freq=50  Vinit=[0, 0]  Iinit=[0, 0]  Ts=1/fsw
      settings: LibrarySourceBlock=|
      | sps_lib/Sensors and Measurements/Power
      | (Positive-Sequence)
  Scope{,1..3} (4 alike) : Scope  NumInputPorts=2
  Scope{4,6..8} (4 alike) : Scope
  Scope5 : Scope  NumInputPorts=3
  Sum{,1..2,4,6} (5 alike) : Sum  Inputs=|+-
  Sum3 : Sum  Inputs=+|+|-
  Sum5 : Sum  Inputs=+|+
  Sum7 : Sum  Inputs=+|+|+
  dq0 to abc : spsdq0toabcLib/dq0 to abc  Alignment=90 degrees behind phase A axis
  gate : Outport
  wires:
  Constant/1 -> Mux/3
  PID Controller2/1 -> Sum5/2
  wt/1 -> dq0 to abc/2
  Mux/1 -> dq0 to abc/1
  Ud_ref/1 -> Scope/1, Sum/1
  Iq/1 -> Gain1/1, Sum6/2, Scope3/2
  Uq/1 -> Sum4/2, Scope1/2, Sum7/3, Gain3/1
  Sum3/1 -> Mux/1
  Sum5/1 -> Scope3/1, Sum6/1  "iq_ref"
  Sum2/1 -> PID Controller1/1
  Sum/1 -> PID Controller/1
  Sum7/1 -> Mux/2
  PID Controller1/1 -> Sum3/2  "Idef"
  Gain/1 -> Sum5/1
  Uq_ref/1 -> Scope1/1, Sum4/1
  Ud/1 -> Scope/2, Sum/2, Sum3/1, Gain/1
  Sum6/1 -> PID Controller3/1
  Sum4/1 -> PID Controller2/1
  Id/1 -> Gain4/1, Sum2/2, Scope2/2
  PID Controller3/1 -> Sum7/2  "Idef"
  PWM Generator (2-Level)/1 -> gate/1
  dq0 to abc/1 -> Gain2/1
  Gain2/1 -> Scope4/1, PWM Generator (2-Level)/1
  PID Controller/1 -> Sum1/1
  Gain3/1 -> Sum1/2
  Sum1/1 -> Scope2/1, Sum2/1
  Gain1/1 -> Sum3/3
  Gain4/1 -> Sum7/1
  PLL (3ph)/1 -> Scope8/1
  [Iabc] -> Power (Positive-Sequence)/2
  Demux3/1 -> Scope5/1
  Demux3/2 -> Scope5/2
  Power (Positive-Sequence)/1 -> Display1/1, Scope6/1
  [Uabc] -> PLL (3ph)/1, Power (Positive-Sequence)/1, Demux3/1
  Power (Positive-Sequence)/2 -> Display2/1, Scope7/1
  Demux3/3 -> Scope5/3

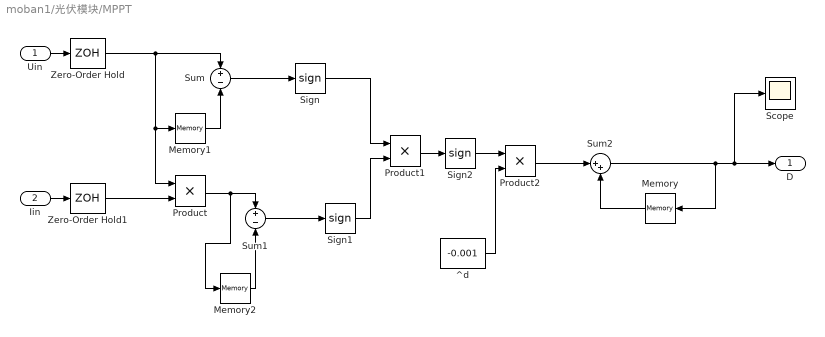
== system moban1/光伏模块/MPPT ==
  Uin : Inport
  Iin : Inport  Port=2
  Memory : Memory  InitialCondition=0.85
  Memory1 : Memory  InitialCondition=0.5
  Memory2 : Memory  InitialCondition=10
  Product : Product  RndMeth=Zero
  Product1 : Product  RndMeth=Zero
  Product2 : Product  RndMeth=Zero
  Scope : Scope
  Sign : Signum  SampleTime=0
  Sign1 : Signum  SampleTime=0
  Sign2 : Signum
  Sum : Sum  Inputs=+-
  Sum1 : Sum  Inputs=+-
  Sum2 : Sum  Inputs=|++
  Zero-Order Hold : ZeroOrderHold  SampleTime=1e-4
  Zero-Order Hold1 : ZeroOrderHold  SampleTime=1e-4
  ^d : Constant  Value=-0.001
  D : Outport  VectorParamsAs1DForOutWhenUnconnected=off
  wires:
  Zero-Order Hold/1 -> Sum/1, Memory1/1, Product/1
  Sum/1 -> Sign/1
  Memory1/1 -> Sum/2
  Zero-Order Hold1/1 -> Product/2
  Product/1 -> Sum1/1, Memory2/1
  Sum1/1 -> Sign1/1
  Memory2/1 -> Sum1/2
  Sign1/1 -> Product1/2
  Sign/1 -> Product1/1
  ^d/1 -> Product2/2
  Sum2/1 -> Memory/1, Scope/1, D/1
  Memory/1 -> Sum2/2
  Uin/1 -> Zero-Order Hold/1
  Iin/1 -> Zero-Order Hold1/1
  Sign2/1 -> Product2/1
  Product1/1 -> Sign2/1
  Product2/1 -> Sum2/1

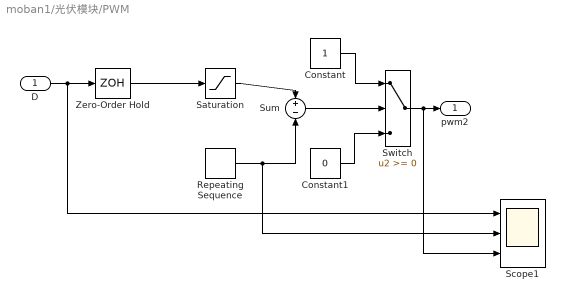
== system moban1/光伏模块/PWM ==
  D : Inport
  Constant : Constant
  Constant1 : Constant  Value=0
  Repeating Sequence : simulink/Sources/Repeating Sequence  rep_seq_t=[0 1e-4]  rep_seq_y=[0 1]
  Saturation : Saturate  UpperLimit=1  LowerLimit=-1  SampleTime=0
  Scope1 : Scope  NumInputPorts=3
  Sum : Sum  Inputs=+-
  Switch : Switch  SaturateOnIntegerOverflow=off  InputSameDT=off
  Zero-Order Hold : ZeroOrderHold  SampleTime=1e-4
  pwm2 : Outport  VectorParamsAs1DForOutWhenUnconnected=off
  wires:
  D/1 -> Scope1/1, Zero-Order Hold/1
  Zero-Order Hold/1 -> Saturation/1
  Saturation/1 -> Sum/1
  Repeating Sequence/1 -> Scope1/2, Sum/2
  Sum/1 -> Switch/2
  Constant/1 -> Switch/1
  Constant1/1 -> Switch/3
  Switch/1 -> Scope1/3, pwm2/1

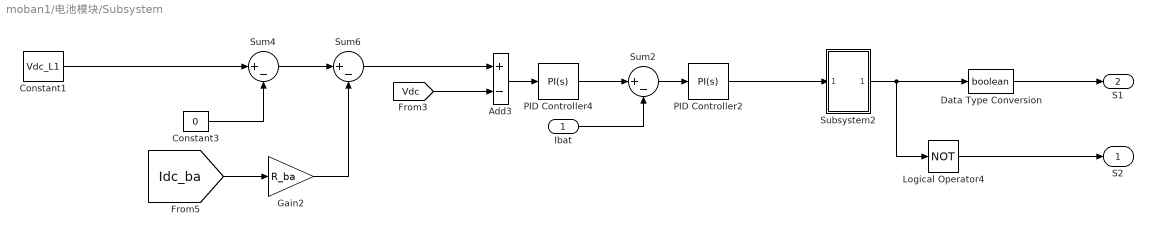
== system moban1/电池模块/Subsystem ==
  Ibat : Inport
  Add3 : Sum  Inputs=+-
  Constant1 : Constant  Value=Vdc_L1
  Constant3 : Constant  Value=0
  Data Type Conversion : DataTypeConversion  OutDataTypeStr=boolean  SaturateOnIntegerOverflow=off  RndMeth=Floor
  Gain2 : Gain  Gain=R_ba
  Logical Operator4 : Logic  Operator=NOT  AllPortsSameDT=off  OutDataTypeStr=boolean
  PID Controller2 : slpidlib/PID Controller  Controller=PI  Form=Parallel  TimeDomain=Continuous-time  UseExternalTs=off  SampleTime=-1  IntegratorMethod=Forward Euler  FilterMethod=Forward Euler  ControllerParametersSource=internal  P=1  I=1  UseKiTs=off  D=0  N=100  UseFilter=on  TunerSelectOption=Transfer Function Based (PID Tuner App)  InitialConditionSource=internal  InitialConditionForIntegrator=0  InitialConditionForFilter=0  DifferentiatorICPrevScaledInput=0  ExternalReset=none  TrackingMode=off  Kt=1  LimitOutput=off  SatLimitsSource=internal  UpperSaturationLimit=inf  LowerSaturationLimit=-inf  LinearizeAsGain=on  AntiWindupMode=none  Kb=1  LimitIntegrator=off  UpperIntegratorSaturationLimit=inf  LowerIntegratorSaturationLimit=-inf  POutMin=[]  POutMax=[]  IOutMin=[]  IOutMax=[]  DOutMin=[]  DOutMax=[]  NOutMin=[]  NOutMax=[]  SumOutMin=[]  SumOutMax=[]  SaturationOutMin=[]  SaturationOutMax=[]  PParamMin=[]  PParamMax=[]  IParamMin=[]  IParamMax=[]  DParamMin=[]  DParamMax=[]  NParamMin=[]  NParamMax=[]  KbParamMin=[]  KbParamMax=[]  KtParamMin=[]  KtParamMax=[]  KbOutMin=[]  KbOutMax=[]  KtOutMin=[]  KtOutMax=[]  IntegratorOutMin=[]  IntegratorOutMax=[]  FilterOutMin=[]  FilterOutMax=[]  SumI1OutMin=[]  SumI1OutMax=[]  SumI2OutMin=[]  SumI2OutMax=[]  SumI3OutMin=[]  SumI3OutMax=[]  SumI4OutMin=[]  SumI4OutMax=[]  SumDOutMin=[]  SumDOutMax=[]  DifferentiatorOutMin=[]  DifferentiatorOutMax=[]  FilterDiffOutCoefMin=[]  FilterDiffOutCoefMax=[]  ReciprocalOutMin=[]  ReciprocalOutMax=[]  SumDenOutMin=[]  SumDenOutMax=[]  SumNumOutMin=[]  SumNumOutMax=[]  DivideOutMin=[]  DivideOutMax=[]  UdiffTsProdOutMin=[]  UdiffTsProdOutMax=[]  NTsProdOutMin=[]  NTsProdOutMax=[]  UintegralTsProdOutMin=[]  UintegralTsProdOutMax=[]  UngainTsProdOutMin=[]  UngainTsProdOutMax=[]  ClampingZeroOutDataTypeStr=Inherit: Inherit via back propagation  ClampingZeroOutMin=[]  ClampingZeroOutMax=[]  FilterDenConstantOutDataTypeStr=Inherit: Inherit via back propagation  FilterDenConstantOutMin=[]  FilterDenConstantOutMax=[]  PCopyOutDataTypeStr=Inherit: Inherit via back propagation  PCopyOutMin=[]  PCopyOutMax=[]  NCopyOutDataTypeStr=Inherit: Inherit via back propagation  NCopyOutMin=[]  NCopyOutMax=[]  IntegratorContinuousStateAttributes=''  IntegratorStateMustResolveToSignalObject=off  IntegratorRTWStateStorageClass=Auto  FilterContinuousStateAttributes=''  FilterStateMustResolveToSignalObject=off  FilterRTWStateStorageClass=Auto  ParallelPVariant=InternalParameters  IdealPVariant=Disabled  IVariant=InternalParameters  DVariant=Disabled  IntegratorVariant=Continuous  SatVariant=Disabled  AWVariant=Passthrough  PCopyVariant=Disabled  TRVariant=Disabled  FdbkBlocksVariant=Forward  IdealPFdbkVariant=Disabled  SatFdbkVariant=Disabled  DerivativeFilterVariant=Disabled  NVariant=Disabled  NCopyVariant=Disabled_SignalSpec  FilterICVariant=Disabled  IntegratorICVariant=InternalICs  ExternalResetVariant=Disabled  TRSumVariant=Passthrough  SumFdbkVariant=Disabled  SumVariant=Sum_PI  TsampFilterVariant=InternalTs  TsampNgainVariant=Passthrough  TsampIntegralVariant=Passthrough  ExternalSaturationOutDataTypeStr=Inherit: Same as second input
  PID Controller4 : slpidlib/PID Controller  Controller=PI  Form=Parallel  TimeDomain=Continuous-time  UseExternalTs=off  SampleTime=-1  IntegratorMethod=Forward Euler  FilterMethod=Forward Euler  ControllerParametersSource=internal  P=1  I=20  UseKiTs=off  D=0  N=100  UseFilter=on  TunerSelectOption=Transfer Function Based (PID Tuner App)  InitialConditionSource=internal  InitialConditionForIntegrator=0  InitialConditionForFilter=0  DifferentiatorICPrevScaledInput=0  ExternalReset=none  TrackingMode=off  Kt=1  LimitOutput=on  SatLimitsSource=internal  UpperSaturationLimit=Iba_max  LowerSaturationLimit=-Iba_max  LinearizeAsGain=on  AntiWindupMode=none  Kb=1  LimitIntegrator=off  UpperIntegratorSaturationLimit=inf  LowerIntegratorSaturationLimit=-inf  POutMin=[]  POutMax=[]  IOutMin=[]  IOutMax=[]  DOutMin=[]  DOutMax=[]  NOutMin=[]  NOutMax=[]  SumOutMin=[]  SumOutMax=[]  SaturationOutMin=[]  SaturationOutMax=[]  PParamMin=[]  PParamMax=[]  IParamMin=[]  IParamMax=[]  DParamMin=[]  DParamMax=[]  NParamMin=[]  NParamMax=[]  KbParamMin=[]  KbParamMax=[]  KtParamMin=[]  KtParamMax=[]  KbOutMin=[]  KbOutMax=[]  KtOutMin=[]  KtOutMax=[]  IntegratorOutMin=[]  IntegratorOutMax=[]  FilterOutMin=[]  FilterOutMax=[]  SumI1OutMin=[]  SumI1OutMax=[]  SumI2OutMin=[]  SumI2OutMax=[]  SumI3OutMin=[]  SumI3OutMax=[]  SumI4OutMin=[]  SumI4OutMax=[]  SumDOutMin=[]  SumDOutMax=[]  DifferentiatorOutMin=[]  DifferentiatorOutMax=[]  FilterDiffOutCoefMin=[]  FilterDiffOutCoefMax=[]  ReciprocalOutMin=[]  ReciprocalOutMax=[]  SumDenOutMin=[]  SumDenOutMax=[]  SumNumOutMin=[]  SumNumOutMax=[]  DivideOutMin=[]  DivideOutMax=[]  UdiffTsProdOutMin=[]  UdiffTsProdOutMax=[]  NTsProdOutMin=[]  NTsProdOutMax=[]  UintegralTsProdOutMin=[]  UintegralTsProdOutMax=[]  UngainTsProdOutMin=[]  UngainTsProdOutMax=[]  ClampingZeroOutDataTypeStr=Inherit: Inherit via back propagation  ClampingZeroOutMin=[]  ClampingZeroOutMax=[]  FilterDenConstantOutDataTypeStr=Inherit: Inherit via back propagation  FilterDenConstantOutMin=[]  FilterDenConstantOutMax=[]  PCopyOutDataTypeStr=Inherit: Inherit via back propagation  PCopyOutMin=[]  PCopyOutMax=[]  NCopyOutDataTypeStr=Inherit: Inherit via back propagation  NCopyOutMin=[]  NCopyOutMax=[]  IntegratorContinuousStateAttributes=''  IntegratorStateMustResolveToSignalObject=off  IntegratorRTWStateStorageClass=Auto  FilterContinuousStateAttributes=''  FilterStateMustResolveToSignalObject=off  FilterRTWStateStorageClass=Auto  ParallelPVariant=InternalParameters  IdealPVariant=Disabled  IVariant=InternalParameters  DVariant=Disabled  IntegratorVariant=Continuous  SatVariant=Enabled  AWVariant=Passthrough  PCopyVariant=Disabled  TRVariant=Disabled  FdbkBlocksVariant=Forward  IdealPFdbkVariant=Disabled  SatFdbkVariant=Disabled  DerivativeFilterVariant=Disabled  NVariant=Disabled  NCopyVariant=Disabled_SignalSpec  FilterICVariant=Disabled  IntegratorICVariant=InternalICs  ExternalResetVariant=Disabled  TRSumVariant=Passthrough  SumFdbkVariant=Disabled  SumVariant=Sum_PI  TsampFilterVariant=InternalTs  TsampNgainVariant=Passthrough  TsampIntegralVariant=Passthrough  ExternalSaturationOutDataTypeStr=Inherit: Same as second input
  Subsystem2 : Subsystem
  Sum2 : Sum  Inputs=|+-
  Sum4 : Sum  Inputs=|+-
  Sum6 : Sum  Inputs=|+-
  S2 : Outport  VectorParamsAs1DForOutWhenUnconnected=off
  S1 : Outport  Port=2  VectorParamsAs1DForOutWhenUnconnected=off
  wires:
  Data Type Conversion/1 -> S1/1
  Ibat/1 -> Sum2/2
  Constant1/1 -> Sum4/1
  Add3/1 -> PID Controller4/1
  Sum4/1 -> Sum6/1
  Gain2/1 -> Sum6/2
  PID Controller2/1 -> Subsystem2/1(In1)
  [Idc_ba] -> Gain2/1
  Sum2/1 -> PID Controller2/1
  [Vdc] -> Add3/2
  Subsystem2/1(Out1) -> Data Type Conversion/1, Logical Operator4/1
  Sum6/1 -> Add3/1
  PID Controller4/1 -> Sum2/1
  Logical Operator4/1 -> S2/1
  Constant3/1 -> Sum4/2

== system moban1/交流测/  /Signal Builder ==
  Demux : Demux  Tag=STV Demux  Outputs=1
      settings: DisplayOption=none
  FromWs : FromWorkspace  Tag=STV FromWs  VariableName=tuvar
      SigBuilderData=|
      | common.afterFinalStr = 'Extrapolate'
      | common.sampleTime = 0
      | dataSet.timeRange = [0 10]
      | dataSet.name = 'Group 1'
      | sbobj.Groups.Name = 'Group 1'
      | sbobj.Groups.Signals.Name = 'Signal 1'
      | sbobj.Groups.Signals.XData = [0 1 1 1.5 1.5 10]
      | sbobj.Groups.Signals.YData = [0 0 0.99 0.99 1 0]
  Signal 1 : Outport  Tag=STV Outport
  wires:
  Demux/1 -> Signal 1/1
  FromWs/1 -> Demux/1

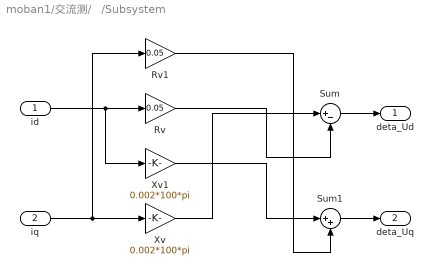
== system moban1/交流测/   /Subsystem ==
  id : Inport
  iq : Inport  Port=2
  Rv : Gain  Gain=0.05
  Rv1 : Gain  Gain=0.05
  Sum : Sum  Inputs=|+-
  Sum1 : Sum  Inputs=|++
  Xv : Gain  Gain=0.002*100*pi
  Xv1 : Gain  Gain=0.002*100*pi
  deta_Ud : Outport
  deta_Uq : Outport  Port=2
  wires:
  Sum/1 -> deta_Ud/1
  Sum1/1 -> deta_Uq/1
  id/1 -> Xv1/1, Rv/1
  Rv/1 -> Sum/2
  iq/1 -> Rv1/1, Xv/1
  Xv/1 -> Sum/1
  Xv1/1 -> Sum1/1
  Rv1/1 -> Sum1/2
